simulink model "LAB1_1_mot"  (R2024b)
settings: Solver=ode3  StartTime=0.0  StopTime=10  FixedStep=0.001  RelTol=1e-3
values from neighbouring files (symbols this model uses):
  BEMF_comp = (gbox.N*mot.Ke)/drv.dcgain    [LAB1_Corretto.m]
  Fri_comp = (Req)/(drv.dcgain*mot.Kt*gbox.N)    [LAB1_Corretto.m]
  In_comp = (gbox.N*Req*Jeq)/(drv.dcgain*mot.Kt)    [LAB1_Corretto.m]
  Kw = 1/Tw    (= 33.3333333333)    [LAB1_Corretto.m]
  om_comp = (gbox.N^2* Beq)    [LAB1_Corretto.m]
  Tausf = tau_sf_est    [LAB1_Corretto.m]    (also in LAB1_GIOI.m)
undefined symbols (not defined in the file or in its folder): daq, degs2rpm, den_Hi, den_Hw, Kd, Ki, Kp, mot, National_Instruments, num_Hi, num_Hw, PCI, sens, Tl
libraries: sldrtlib x3, simulink x1
settings Model: SimulationMode=external  ExtModeTrigDuration=100001  Creator=delpratogi  LastModifiedBy=delpratogi
settings DataIOCC: ReturnWorkspaceOutputs=off
settings HardwareCC: ProdBitPerLong=64  ProdHWDeviceType=Intel->x86-64 (Linux 64)
settings RTWCC: Description=Simulink Desktop Real-Time  SystemTargetFile=sldrt.tlc  TemplateMakefile=sldrt.tmf  RTWCompilerOptimization=on
settings CodeAppCC: MaxIdLength=95
settings SimulinkDesktopRealTimeCC: TargetLibSuffix=_sldrt.a  TargetPreCompLibLocation=C:\Program Files\MATLAB\R2024b\toolbox\sldrt\lib\win64  ParMdlRefBuildCompliant=on

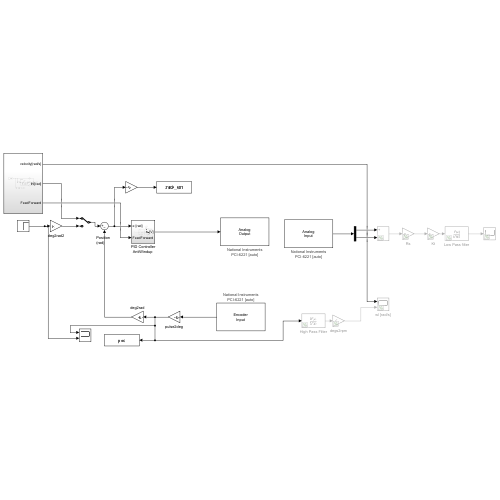
[thumbnail: Simulink's stored preview of the top-level diagram]
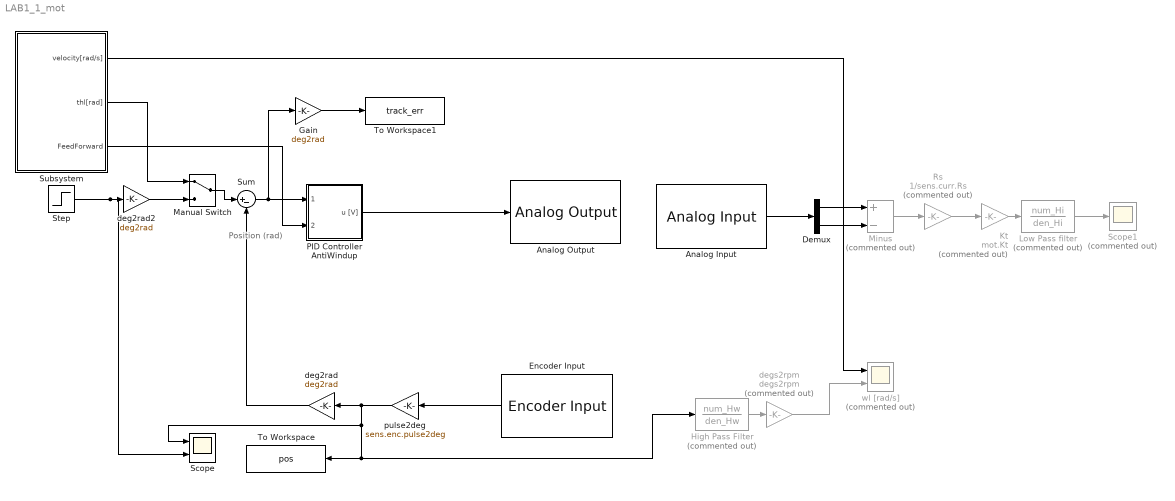
== system LAB1_1_mot ==
  note: Position
      | (rad)
  Analog Input : sldrtlib/Analog Input  SampleTime=0.001  MaxMissedTicks=10  ShowMissedTicks=off  YieldWhenWaiting=off  DrvName=National_Instruments/PCI-6221  DrvAddress=4294967295  DrvOptions=[0 0 0 2 0]  Channels=[1,2]  RangeMode=1  VoltRange=1  DataType=1
      settings: AttributesFormatString=National Instruments\nPCI-6221 [auto]
  Analog Output : sldrtlib/Analog Output  SampleTime=0.001  MaxMissedTicks=10  ShowMissedTicks=off  YieldWhenWaiting=off  DrvName=National_Instruments/PCI-6221  DrvAddress=4294967295  DrvOptions=[0 0 0 2 0]  Channels=1  RangeMode=1  VoltRange=1  InitialValue=0  FinalValue=0
      settings: AttributesFormatString=National Instruments\nPCI-6221 [auto]
  Demux : Demux  Outputs=2
  Encoder Input : sldrtlib/Encoder Input  SampleTime=0.001  MaxMissedTicks=10  ShowMissedTicks=off  YieldWhenWaiting=off  DrvName=National_Instruments/PCI-6221  DrvAddress=4294967295  DrvOptions=[0 0 0 2 0]  Channels=1  QuadMode=3  IndexPulse=1  InputFilter=Inf  DataType=1
      settings: AttributesFormatString=National Instruments\nPCI-6221 [auto]
  Gain : Gain  Gain=deg2rad
  High Pass Filter : TransferFcn  Commented=on  Numerator=num_Hw  Denominator=den_Hw
  Kt : Gain  Commented=on  Gain=mot.Kt
  Low Pass filter : TransferFcn  Commented=on  Numerator=num_Hi  Denominator=den_Hi
  Manual Switch : ManualSwitch
  Minus : Sum  Commented=on  Inputs=+-
  "PID Controller AntiWindup " : Subsystem
  Rs : Gain  Commented=on  Gain=1/sens.curr.Rs
  Scope : Scope  NumInputPorts=2
  Scope1 : Scope  Commented=on
  Step : Step  Time=0  After=360  SampleTime=0
  Subsystem : Subsystem
  Sum : Sum  Inputs=|+-
  To Workspace : ToWorkspace  VariableName=pos  SaveFormat=Structure With Time  SampleTime=-1
  To Workspace1 : ToWorkspace  VariableName=track_err  SaveFormat=Structure With Time  SampleTime=-1
  deg2rad : Gain  Gain=deg2rad
  deg2rad2 : Gain  Gain=deg2rad
  degs2rpm : Gain  Commented=on  Gain=degs2rpm
  pulse2deg : Gain  Gain=sens.enc.pulse2deg
  wl [rad/s] : Scope  Commented=on  NumInputPorts=2
  wires:
  Analog Input/1 -> Demux/1
  Demux/1 -> Minus/1
  Encoder Input/1 -> pulse2deg/1
  Minus/1 -> Rs/1
  Demux/2 -> Minus/2
  Rs/1 -> Kt/1
  Low Pass filter/1 -> Scope1/1
  Kt/1 -> Low Pass filter/1
  pulse2deg/1 -> To Workspace/1, High Pass Filter/1, Scope/1, deg2rad/1
  degs2rpm/1 -> wl [rad/s]/2
  High Pass Filter/1 -> degs2rpm/1
  "PID Controller AntiWindup "/1(u [V]) -> Analog Output/1
  Sum/1 -> Gain/1, "PID Controller AntiWindup "/1(e [rad])
  deg2rad/1 -> Sum/2
  Subsystem/3(FeedForward) -> "PID Controller AntiWindup "/2(FeedForward)
  Subsystem/1(velocity[rad/s]) -> wl [rad/s]/1
  Step/1 -> Scope/2, deg2rad2/1
  Gain/1 -> To Workspace1/1
  deg2rad2/1 -> Manual Switch/2
  Manual Switch/1 -> Sum/1
  Subsystem/2(thl[rad]) -> Manual Switch/1

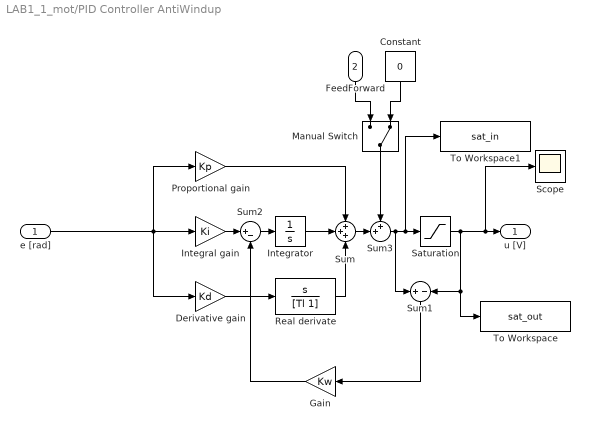
== system LAB1_1_mot/PID Controller AntiWindup  ==
  e [rad] : Inport
  FeedForward : Inport  Port=2
  Constant : Constant  Value=0
  Derivative gain : Gain  Gain=Kd
  Gain : Gain  Gain=Kw
  "Integral gain " : Gain  Gain=Ki
  Integrator : Integrator
  Manual Switch : ManualSwitch  CurrentSetting=0
  Proportional gain : Gain  Gain=Kp
  Real derivate : TransferFcn  Numerator=[1 0]  Denominator=[Tl 1]
  Saturation : Saturate  UpperLimit=daq.dac.fs  LowerLimit=-daq.dac.fs
  Scope : Scope
  Sum : Sum  Inputs=+++
  Sum1 : Sum  Inputs=+|-
  Sum2 : Sum  Inputs=|+-
  Sum3 : Sum  Inputs=++|
  To Workspace : ToWorkspace  VariableName=sat_out  SaveFormat=Structure With Time  SampleTime=-1
  To Workspace1 : ToWorkspace  VariableName=sat_in  SaveFormat=Structure With Time  SampleTime=-1
  u [V] : Outport
  wires:
  Real derivate/1 -> Sum/3
  Integrator/1 -> Sum/2
  e [rad]/1 -> Proportional gain/1, Derivative gain/1, "Integral gain "/1
  Proportional gain/1 -> Sum/1
  Derivative gain/1 -> Real derivate/1
  Saturation/1 -> To Workspace/1, Sum1/2, Scope/1, u [V]/1
  Sum1/1 -> Gain/1
  "Integral gain "/1 -> Sum2/1
  Sum2/1 -> Integrator/1
  Gain/1 -> Sum2/2
  Sum3/1 -> Sum1/1, To Workspace1/1, Saturation/1
  Sum/1 -> Sum3/2
  FeedForward/1 -> Manual Switch/1
  Constant/1 -> Manual Switch/2
  Manual Switch/1 -> Sum3/1

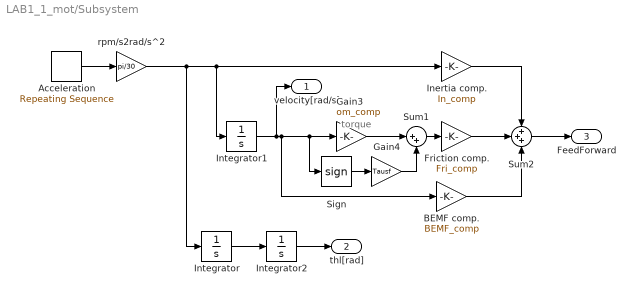
== system LAB1_1_mot/Subsystem ==
  note: torque
  Acceleration : simulink/Sources/Repeating Sequence  rep_seq_t=[0, 0.5, 0.50001, 1, 1.0001, 2, 2.0001, 2.5, 2.50001, 3]  rep_seq_y=[900, 900, 0, 0, -900, -900, 0, 0, 900, 900]
  BEMF comp. : Gain  Gain=BEMF_comp
  Friction comp. : Gain  Gain=Fri_comp
  Gain3 : Gain  Gain=om_comp
  Gain4 : Gain  Gain=Tausf
  Inertia comp. : Gain  Gain=In_comp
  Integrator : Integrator
  Integrator1 : Integrator
  Integrator2 : Integrator
  Sign : Signum  ZeroCross=off
  Sum1 : Sum  Inputs=|++
  Sum2 : Sum  Inputs=+++
  rpm/s2rad/s^2 : Gain  Gain=pi/30
  velocity[rad/s] : Outport
  thl[rad] : Outport  Port=2
  FeedForward : Outport  Port=3
  wires:
  Integrator/1 -> Integrator2/1
  Sign/1 -> Gain4/1
  Acceleration/1 -> rpm/s2rad/s^2/1
  Gain4/1 -> Sum1/2
  Integrator1/1 -> velocity[rad/s]/1, BEMF comp./1, Sign/1, Gain3/1
  Gain3/1 -> Sum1/1
  Sum1/1 -> Friction comp./1
  rpm/s2rad/s^2/1 -> Integrator/1, Integrator1/1, Inertia comp./1
  Inertia comp./1 -> Sum2/1
  Friction comp./1 -> Sum2/2
  BEMF comp./1 -> Sum2/3
  Integrator2/1 -> thl[rad]/1
  Sum2/1 -> FeedForward/1
